simulink model "EOM_solver_matthias"  (R2023b)
settings: Solver=ode45  StartTime=0.0  StopTime=2  FixedStep=0.1  RelTol=1e-3
values from neighbouring files (symbols this model uses):
  a_c = 0    [EOM_input.m]    (also in Mechatronics.m)
  b_c = 0    [EOM_input.m]    (also in Mechatronics.m)
  M = M_a + M_rb    [EOM_input.m]    (also in Mechatronics (1).m; Mechatronics.m)
  speed_c = 0.2    [EOM_input.m]    (also in Mechatronics.m = 2)
  tau = [tau_u;tau_v;tau_r]    [EOM_input.m]    (also in Mechatronics (1).m; Mechatronics.m)
  tau_e = [0; 0; 0]    [EOM_input.m]    (also in Mechatronics (1).m = 0; Mechatronics.m = [0 0 0])
libraries: matrix_library x4
settings Model: Creator=chris  LastModifiedBy=chris

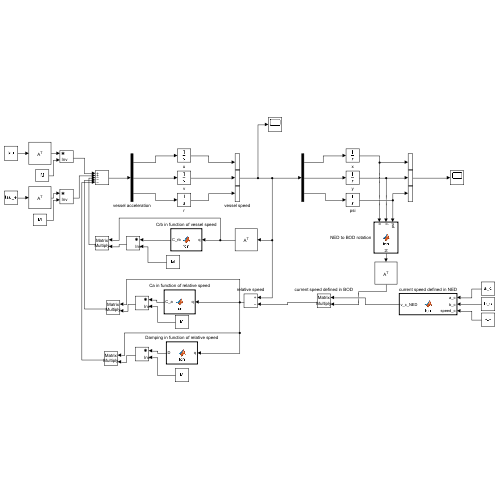
[thumbnail: Simulink's stored preview of the top-level diagram]
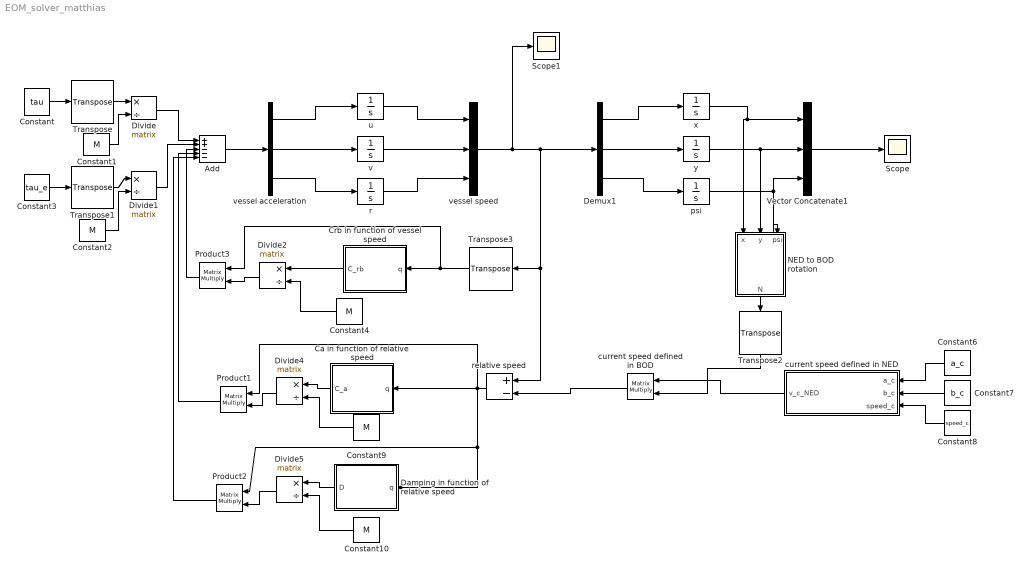
== system EOM_solver_matthias ==
  Add : Sum  Inputs=++---
  Ca in function of relative speed : MATLAB Function  TreatAsAtomicUnit=on
  Constant : Constant  Value=tau
  Constant{1..2,4,9..10} (5 alike) : Constant  Value=M
  Constant3 : Constant  Value=tau_e
  Constant6 : Constant  Value=a_c
  Constant7 : Constant  Value=b_c
  Constant8 : Constant  Value=speed_c
  Crb in function of vessel speed : MATLAB Function  TreatAsAtomicUnit=on
  Damping in function of relative speed : MATLAB Function  TreatAsAtomicUnit=on
  Demux1 : Demux  Outputs=3
  Divide{,1..2,4..5} (5 alike) : Product  Inputs=*/  Multiplication=Matrix(*)
  NED to BOD rotation : MATLAB Function  TreatAsAtomicUnit=on
  Product1 : Product  Multiplication=Matrix(*)
  Product2 : Product  Multiplication=Matrix(*)
  Product3 : Product  Multiplication=Matrix(*)
  Scope : Scope
  Scope1 : Scope
  Transpose{,1..3} (4 alike) : matrix_library/Transpose
  Vector Concatenate1 : Concatenate  NumInputs=3
  current speed defined in BOD : Product  Multiplication=Matrix(*)
  current speed defined in NED : MATLAB Function  TreatAsAtomicUnit=on
  psi : Integrator
  r : Integrator
  relative speed : Sum  Inputs=+-
  u : Integrator
  v : Integrator
  vessel acceleration : Demux  Outputs=3
  vessel speed : Concatenate  NumInputs=3
  x : Integrator
  y : Integrator
  wires:
  Constant/1 -> Transpose/1
  Constant1/1 -> Divide/2
  Constant3/1 -> Transpose1/1
  Divide/1 -> Add/1
  Divide1/1 -> Add/2
  Add/1 -> vessel acceleration/1
  vessel acceleration/1 -> u/1
  vessel acceleration/2 -> v/1
  vessel acceleration/3 -> r/1
  u/1 -> vessel speed/1
  v/1 -> vessel speed/2
  r/1 -> vessel speed/3
  vessel speed/1 -> Scope1/1, relative speed/1, Transpose3/1, Demux1/1
  Crb in function of vessel speed/1(C_rb) -> Divide2/1
  Transpose/1 -> Divide/1
  Transpose1/1 -> Divide1/1
  Constant2/1 -> Divide1/2
  Constant4/1 -> Divide2/2
  Demux1/1 -> x/1
  Demux1/2 -> y/1
  Demux1/3 -> psi/1
  y/1 -> Vector Concatenate1/2, NED to BOD rotation/2(y)
  x/1 -> Vector Concatenate1/1, NED to BOD rotation/1(x)
  psi/1 -> Vector Concatenate1/3, NED to BOD rotation/3(psi)
  NED to BOD rotation/1(N) -> Transpose2/1
  Constant7/1 -> current speed defined in NED/2(b_c)
  Constant6/1 -> current speed defined in NED/1(a_c)
  Constant8/1 -> current speed defined in NED/3(speed_c)
  current speed defined in BOD/1 -> relative speed/2
  relative speed/1 -> Product1/1, Ca in function of relative speed/1(q), Damping in function of relative speed/1(q), Product2/1
  Ca in function of relative speed/1(C_a) -> Divide4/1
  Constant9/1 -> Divide4/2
  Damping in function of relative speed/1(D) -> Divide5/1
  Constant10/1 -> Divide5/2
  Product1/1 -> Add/4
  Product2/1 -> Add/5
  Vector Concatenate1/1 -> Scope/1
  Divide4/1 -> Product1/2
  Divide5/1 -> Product2/2
  Transpose3/1 -> Product3/1, Crb in function of vessel speed/1(q)
  Divide2/1 -> Product3/2
  Product3/1 -> Add/3
  current speed defined in NED/1(v_c_NED) -> current speed defined in BOD/1
  Transpose2/1 -> current speed defined in BOD/2

== matlab function EOM_solver_matthias/Crb in function of vessel speed ==
  data: q input; C_rb output
function C_rb = fcn(q)
u = q(1);
v = q(2);
r = q(3);

x_g = 0; % body fixed reference system located at COG
y_g = 0;
m = 18; % Mass

C_rb = [0,0, -m*(x_g*r+v);
        0,0, -m*(y_g*r-u);
        m*(x_g*r + v), m*(y_g*r- u),0];

== matlab function EOM_solver_matthias/current speed defined in NED ==
  data: a_c input; v_c_NED output; b_c input; speed_c input
function v_c_NED = fcn(a_c, b_c, speed_c)
v_c_NED = [speed_c*cos(a_c)*cos(b_c) speed_c*sin(b_c) speed_c*sin(a_c)*cos(b_c)];

== matlab function EOM_solver_matthias/NED to BOD rotation ==
  data: x input; N output; y input; psi input
function N = fcn(x, y, psi)
N = [cos(psi) -sin(psi) 0; sin(psi) cos(psi) 0; 0 0 1];

== matlab function EOM_solver_matthias/Ca in function of relative speed ==
  data: q input; C_a output
function C_a = fcn(q)
u = q(1);
v = q(2);
r = q(3);

w = 0; % heave
p = 0; % roll
q = 0; % pitch

X_dotu = 1.2; % all of this given
X_dotv = 0;
X_dotw = 0;
X_dotp = 0;
X_dotq = 0;
X_dotr = 0;

Y_dotu = 0; 
Y_dotv = 66.1; 
Y_dotw = 0;
Y_dotp = 0;
Y_dotq = 0;
Y_dotr = 0;

a_1 = X_dotu*u + X_dotv*v +X_dotw*w + X_dotp*p + X_dotq*q +X_dotr*r;
a_2 = Y_dotu*u + Y_dotv*v +Y_dotw*w + Y_dotp*p + Y_dotq*q +Y_dotr*r;

C_a = [0,   0,   a_2;
       0,   0,  -a_1;
      -a_2, a_1,  0];

== matlab function EOM_solver_matthias/Damping in function of relative speed ==
  data: q input; D output
function D = fcn(q)
u = q(1);
v = q(2);
r = q(3);

d_11 = 0.0069*u^3 - 0.1314*u^2 + 0.8842*u - 2.0431;  %X_drag
d_22 = 0.0289*v^3 - 0.5191*v^2 + 3.3058*v - 2.3601;  %Y_drag
c1 = 122.3;
c2 = 4.8;
L = 0.97;
d_33 = (1/80)*c1*r^3*L^4 + (1/12)*c2*r*L^2;

D = [d_11, 0,   0;
      0,  d_22, 0;
      0,   0,  d_33];
